simulink model "jielie"  (R2014a)
settings: Solver=ode3  StartTime=0.0  StopTime=200  FixedStep=0.05  RelTol=1e-3
libraries: simulink x8
(part 1 of 3)
settings Model: Creator=Uamoo_15  LastModifiedBy=Administrator
settings DebuggingCC: UnderspecifiedInitializationDetection=Classic  StateNameClashWarn=warning

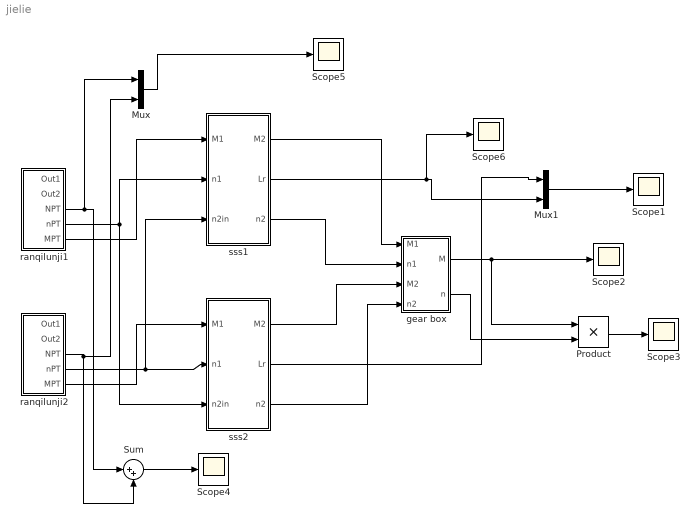
== system jielie ==
  Mux : Mux  Inputs=2
  Mux1 : Mux  Inputs=2
  Product : Product
  Scope{1..6} (6 alike) : Scope
      Scope1 settings: TimeRange=200  YMin=0  YMax=1400  SaveName=ScopeData2
      Scope2 settings: SaveName=ScopeData13
      Scope3 settings: SaveName=ScopeData19
      Scope4 settings: SaveName=ScopeData21
      Scope5 settings: TimeRange=200  YMin=0  YMax=1400  SaveName=ScopeData23
      Scope6 settings: TimeRange=200  YMin=0  YMax=1400  SaveName=ScopeData12
  Sum : Sum  Inputs=|++
  gear box : Subsystem
  ranqilunji1 : Subsystem
  ranqilunji2 : Subsystem
  sss1 : Subsystem
  sss2 : Subsystem
  wires:
  ranqilunji1/4(nPT) -> sss2/3(n2in), sss1/2(n1)
  ranqilunji2/4(nPT) -> sss1/3(n2in), sss2/2(n1)
  ranqilunji1/5(MPT) -> sss1/1(M1)
  ranqilunji2/5(MPT) -> sss2/1(M1)
  sss1/1(M2) -> gear box/1(M1)
  sss2/1(M2) -> gear box/3(M2)
  sss1/3(n2) -> gear box/2(n1)
  sss2/3(n2) -> gear box/4(n2)
  gear box/1(M) -> Product/1, Scope2/1
  gear box/2(n) -> Product/2
  Product/1 -> Scope3/1
  ranqilunji1/3(NPT) -> Mux/1, Sum/1
  ranqilunji2/3(NPT) -> Mux/2, Sum/2
  Sum/1 -> Scope4/1
  Mux/1 -> Scope5/1
  sss1/2(Lr) -> Scope6/1, Mux1/2
  sss2/2(Lr) -> Mux1/1
  Mux1/1 -> Scope1/1

== system jielie/gear box ==
  note: 并车齿轮箱模型
  M1 : Inport
  n1 : Inport  Port=2
  M2 : Inport  Port=3
  n2 : Inport  Port=4
  Add : Sum
  Fcn : Fcn  Expr=1/u
  Gain : Gain  Gain=1/3.5
  Product : Product
  Product1 : Product
  Product2 : Product
  M : Outport
  n : Outport  Port=2
  wires:
  M1/1 -> Product/1
  n1/1 -> Gain/1, Product/2
  Product/1 -> Add/1
  M2/1 -> Product1/1
  n2/1 -> Product1/2
  Product1/1 -> Add/2
  Gain/1 -> n/1, Fcn/1
  Add/1 -> Product2/1
  Fcn/1 -> Product2/2
  Product2/1 -> M/1

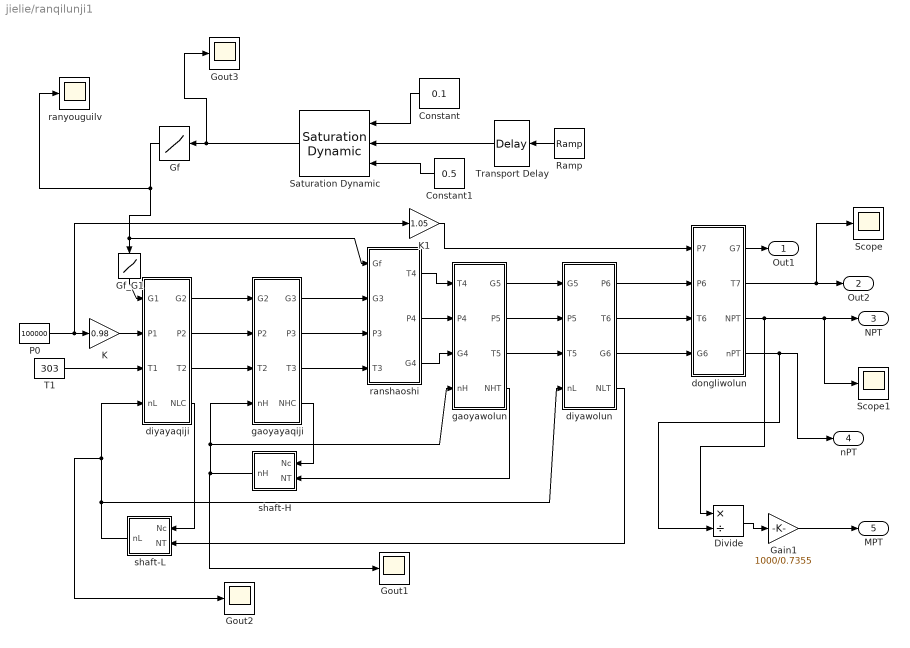
== system jielie/ranqilunji1 ==
  Constant : Constant  Value=0.1
  Constant1 : Constant  Value=0.5
  Divide : Product  Inputs=*/
  Gain1 : Gain  Gain=1000/0.7355
  Gf : Lookup  InputValues=[0,0.03,0.07,0.09,0.11,0.13,0.17,0.2,0.23,0.26,0.28,0.3,0.32,0.34,0.35,0.38,0.4,0.42,0.44,0.47,0.49,0.5,0.52,0.54,0.55,0.59,0.61,0.64,0.66,0.68,0.7,0.72,0.74,0.77,0.81,0.83,0.85,0.88,0.93,0.95,0.97,1]  Table=[0.172,0.236,0.331,0.331,0.366,0.411,0.488,0.536,0.582,0.605,0.644,0.682,0.698,0.728,0.727,0.783,0.783,0.813,0.857,0.886,0.935,0.949,0.95,0.975,0.999,1.022,1.069,1.149,1.153,1.184,1.206,1.233,1.256,1.271,1.325,1.383,1.383,1.439,1.481,1.504,1.52,1.574]
  Gf_G1 : Lookup  InputValues=[0.172,0.236,0.331,0.366,0.411,0.488,0.536,0.582,0.605,0.644,0.682,0.698,0.727,0.728,0.783,0.813,0.857,0.886,0.935,0.949,0.95,0.975,0.999,1.022,1.069,1.149,1.153,1.184,1.206,1.233,1.256,1.271,1.325,1.383,1.439,1.481,1.504,1.52,1.574]  Table="[20.01, 25.93, 38.77,  43.65, 45.94, 51.85, 54.70, 56.85, 59.03, 61.91, 60.44, 61.58, 62.93, 63.04, 65.71,   67.00, 69.52, 70.63, 73.19, 73.46, 73.44, 73.83, 75.62, 76.39, 78.27, 81.17, 81.50, 82.44, 83.44, 84.31, 85.30, 86.17, 87.93, 89.72, 91.51, 93.65, 94.63, 94.92, 97.64]"
  Gout1 : Scope
      settings: TimeRange=10
  Gout2 : Scope
      settings: TimeRange=10  SaveName=ScopeData11
  Gout3 : Scope
      settings: TimeRange=10  SaveName=ScopeData6
  K : Gain  Gain=0.98
  K1 : Gain  Gain=1.05
  P0 : Constant  Value=100000
  Ramp : simulink/Sources/Ramp  slope=1/100  start=0  X0=0.5
  Saturation Dynamic : simulink/Discontinuities/Saturation Dynamic  OutMin=[]  OutMax=[]  OutDataTypeStr=Inherit: Same as second input  OutDataType=fixdt(1, 16)  OutScaling=2^-10  DoSatur=off
  Scope : Scope
      settings: SaveName=ScopeData3
  Scope1 : Scope
      settings: SaveName=ScopeData5
  T1 : Constant  Value=303
  Transport Delay : TransportDelay  DelayTime=40
  diyawolun : Subsystem
  diyayaqiji : Subsystem
  dongliwolun : Subsystem
  gaoyawolun : Subsystem
  gaoyayaqiji : Subsystem
  ranshaoshi : Subsystem
  ranyouguilv : Scope
      settings: TimeRange=10  SaveName=ScopeData8
  shaft-H : Subsystem  mask(rotor module){J=30}
      mask prompts: J "J moment of inertia(Nm)"
      mask help: (pi^2*J*n/900)*(dn/dt)=NT-Nc
  shaft-L : Subsystem  mask(rotor module){J=15}
      mask prompts: J "J moment of inertia(Nm)"
      mask help: (pi^2*J*n/900)*(dn/dt)=NT-Nc
  Out1 : Outport
  Out2 : Outport  Port=2
  NPT : Outport  Port=3
  nPT : Outport  Port=4
  MPT : Outport  Port=5
  wires:
  T1/1 -> diyayaqiji/3(T1)
  K/1 -> diyayaqiji/2(P1)
  diyayaqiji/1(G2) -> gaoyayaqiji/1(G2)
  diyayaqiji/2(P2) -> gaoyayaqiji/2(P2)
  diyayaqiji/3(T2) -> gaoyayaqiji/3(T2)
  gaoyayaqiji/1(G3) -> ranshaoshi/2(G3)
  gaoyayaqiji/2(P3) -> ranshaoshi/3(P3)
  gaoyayaqiji/3(T3) -> ranshaoshi/4(T3)
  gaoyayaqiji/4(NHC) -> shaft-H/1(Nc)
  gaoyawolun/4(NHT) -> shaft-H/2(NT)
  shaft-H/1(nH) -> Gout1/1, gaoyayaqiji/4(nH), gaoyawolun/4(nH)
  diyayaqiji/4(NLC) -> shaft-L/1(Nc)
  diyawolun/4(NLT) -> shaft-L/2(NT)
  Gf_G1/1 -> diyayaqiji/1(G1)
  ranshaoshi/3(G4) -> gaoyawolun/3(G4)
  ranshaoshi/2(P4) -> gaoyawolun/2(P4)
  gaoyawolun/3(T5) -> diyawolun/3(T5)
  gaoyawolun/2(P5) -> diyawolun/2(P5)
  gaoyawolun/1(G5) -> diyawolun/1(G5)
  diyawolun/3(G6) -> dongliwolun/4(G6)
  diyawolun/2(T6) -> dongliwolun/3(T6)
  shaft-L/1(nL) -> diyawolun/4(nL), Gout2/1, diyayaqiji/4(nL)
  diyawolun/1(P6) -> dongliwolun/2(P6)
  P0/1 -> K/1, K1/1
  ranshaoshi/1(T4) -> gaoyawolun/1(T4)
  K1/1 -> dongliwolun/1(P7)
  dongliwolun/1(G7) -> Out1/1
  dongliwolun/2(T7) -> Scope/1, Out2/1
  dongliwolun/3(NPT) -> Divide/1, NPT/1, Scope1/1
  dongliwolun/4(nPT) -> Divide/2, nPT/1
  Constant1/1 -> Saturation Dynamic/3
  Constant/1 -> Saturation Dynamic/1
  Transport Delay/1 -> Saturation Dynamic/2
  Ramp/1 -> Transport Delay/1
  Saturation Dynamic/1 -> Gout3/1, Gf/1
  Gf/1 -> ranyouguilv/1, Gf_G1/1, ranshaoshi/1(Gf)
  Gain1/1 -> MPT/1
  Divide/1 -> Gain1/1

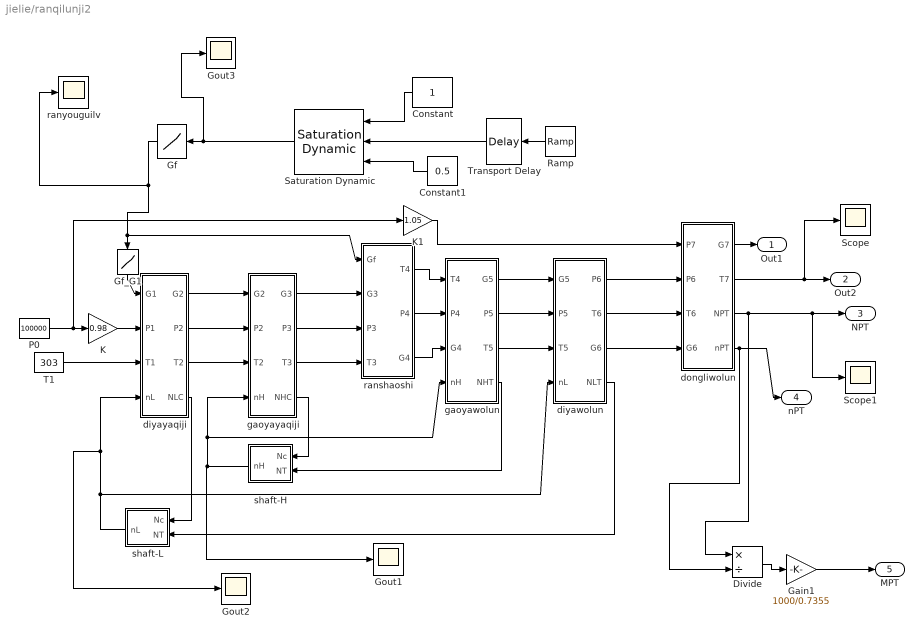
== system jielie/ranqilunji2 ==
  Constant : Constant
  Constant1 : Constant  Value=0.5
  Divide : Product  Inputs=*/
  Gain1 : Gain  Gain=1000/0.7355
  Gf : Lookup  InputValues=[0,0.03,0.07,0.09,0.11,0.13,0.17,0.2,0.23,0.26,0.28,0.3,0.32,0.34,0.35,0.38,0.4,0.42,0.44,0.47,0.49,0.5,0.52,0.54,0.55,0.59,0.61,0.64,0.66,0.68,0.7,0.72,0.74,0.77,0.81,0.83,0.85,0.88,0.93,0.95,0.97,1]  Table=[0.172,0.236,0.331,0.331,0.366,0.411,0.488,0.536,0.582,0.605,0.644,0.682,0.698,0.728,0.727,0.783,0.783,0.813,0.857,0.886,0.935,0.949,0.95,0.975,0.999,1.022,1.069,1.149,1.153,1.184,1.206,1.233,1.256,1.271,1.325,1.383,1.383,1.439,1.481,1.504,1.52,1.574]
  Gf_G1 : Lookup  InputValues=[0.172,0.236,0.331,0.366,0.411,0.488,0.536,0.582,0.605,0.644,0.682,0.698,0.727,0.728,0.783,0.813,0.857,0.886,0.935,0.949,0.95,0.975,0.999,1.022,1.069,1.149,1.153,1.184,1.206,1.233,1.256,1.271,1.325,1.383,1.439,1.481,1.504,1.52,1.574]  Table="[20.01, 25.93, 38.77,  43.65, 45.94, 51.85, 54.70, 56.85, 59.03, 61.91, 60.44, 61.58, 62.93, 63.04, 65.71,   67.00, 69.52, 70.63, 73.19, 73.46, 73.44, 73.83, 75.62, 76.39, 78.27, 81.17, 81.50, 82.44, 83.44, 84.31, 85.30, 86.17, 87.93, 89.72, 91.51, 93.65, 94.63, 94.92, 97.64]"
  Gout1 : Scope
      settings: TimeRange=10
  Gout2 : Scope
      settings: TimeRange=10  SaveName=ScopeData11
  Gout3 : Scope
      settings: TimeRange=10  SaveName=ScopeData6
  K : Gain  Gain=0.98
  K1 : Gain  Gain=1.05
  P0 : Constant  Value=100000
  Ramp : simulink/Sources/Ramp  slope=1/100  start=0  X0=0.5
  Saturation Dynamic : simulink/Discontinuities/Saturation Dynamic  OutMin=[]  OutMax=[]  OutDataTypeStr=Inherit: Same as second input  OutDataType=fixdt(1, 16)  OutScaling=2^-10  DoSatur=off
  Scope : Scope
      settings: SaveName=ScopeData3
  Scope1 : Scope
      settings: SaveName=ScopeData5
  T1 : Constant  Value=303
  Transport Delay : TransportDelay  DelayTime=40
  diyawolun : Subsystem
  diyayaqiji : Subsystem
  dongliwolun : Subsystem
  gaoyawolun : Subsystem
  gaoyayaqiji : Subsystem
  ranshaoshi : Subsystem
  ranyouguilv : Scope
      settings: TimeRange=10  SaveName=ScopeData8
  shaft-H : Subsystem  mask(rotor module){J=30}
      mask prompts: J "J moment of inertia(Nm)"
      mask help: (pi^2*J*n/900)*(dn/dt)=NT-Nc
  shaft-L : Subsystem  mask(rotor module){J=15}
      mask prompts: J "J moment of inertia(Nm)"
      mask help: (pi^2*J*n/900)*(dn/dt)=NT-Nc
  Out1 : Outport
  Out2 : Outport  Port=2
  NPT : Outport  Port=3
  nPT : Outport  Port=4
  MPT : Outport  Port=5
  wires:
  T1/1 -> diyayaqiji/3(T1)
  K/1 -> diyayaqiji/2(P1)
  diyayaqiji/1(G2) -> gaoyayaqiji/1(G2)
  diyayaqiji/2(P2) -> gaoyayaqiji/2(P2)
  diyayaqiji/3(T2) -> gaoyayaqiji/3(T2)
  gaoyayaqiji/1(G3) -> ranshaoshi/2(G3)
  gaoyayaqiji/2(P3) -> ranshaoshi/3(P3)
  gaoyayaqiji/3(T3) -> ranshaoshi/4(T3)
  gaoyayaqiji/4(NHC) -> shaft-H/1(Nc)
  gaoyawolun/4(NHT) -> shaft-H/2(NT)
  shaft-H/1(nH) -> Gout1/1, gaoyayaqiji/4(nH), gaoyawolun/4(nH)
  diyayaqiji/4(NLC) -> shaft-L/1(Nc)
  diyawolun/4(NLT) -> shaft-L/2(NT)
  Gf_G1/1 -> diyayaqiji/1(G1)
  ranshaoshi/3(G4) -> gaoyawolun/3(G4)
  ranshaoshi/2(P4) -> gaoyawolun/2(P4)
  gaoyawolun/3(T5) -> diyawolun/3(T5)
  gaoyawolun/2(P5) -> diyawolun/2(P5)
  gaoyawolun/1(G5) -> diyawolun/1(G5)
  diyawolun/3(G6) -> dongliwolun/4(G6)
  diyawolun/2(T6) -> dongliwolun/3(T6)
  shaft-L/1(nL) -> diyawolun/4(nL), Gout2/1, diyayaqiji/4(nL)
  diyawolun/1(P6) -> dongliwolun/2(P6)
  P0/1 -> K/1, K1/1
  ranshaoshi/1(T4) -> gaoyawolun/1(T4)
  K1/1 -> dongliwolun/1(P7)
  dongliwolun/1(G7) -> Out1/1
  dongliwolun/2(T7) -> Scope/1, Out2/1
  dongliwolun/3(NPT) -> Divide/1, NPT/1, Scope1/1
  dongliwolun/4(nPT) -> Divide/2, nPT/1
  Constant1/1 -> Saturation Dynamic/3
  Constant/1 -> Saturation Dynamic/1
  Transport Delay/1 -> Saturation Dynamic/2
  Ramp/1 -> Transport Delay/1
  Saturation Dynamic/1 -> Gout3/1, Gf/1
  Gf/1 -> ranyouguilv/1, Gf_G1/1, ranshaoshi/1(Gf)
  Gain1/1 -> MPT/1
  Divide/1 -> Gain1/1

== system jielie/sss1 ==
  note: sss离合器模块
  M1 : Inport
  n1 : Inport  Port=2
  n2in : Inport  Port=3
  Add : Sum  Inputs=+-
  Clock : Clock
  Constant : Constant  Value=15
  Fcn : Fcn  Expr=u*pi/30
  Subsystem : Subsystem
  Subsystem1 : Subsystem
  Subsystem2 : Subsystem
  Subsystem3 : Subsystem
  Switch : Switch
  Switch1 : Switch  Threshold=40
  M2 : Outport
  Lr : Outport  Port=2
  n2 : Outport  Port=3
  wires:
  Fcn/1 -> Add/2
  Switch/1 -> n2/1
  M1/1 -> Subsystem3/1(M1)
  Subsystem/1(J1) -> Subsystem3/3(J1)
  Subsystem/2(Jz) -> Subsystem1/2(Jz)
  Subsystem3/1(Mfzf) -> Subsystem1/1(Mfzf)
  Subsystem3/3(C1) -> Subsystem1/3(C1)
  Subsystem1/1(Mr) -> Subsystem2/1(Mr)
  Subsystem1/3(C2) -> Subsystem2/3(C2)
  Subsystem1/2(Lr) -> Switch1/1, Switch/2
  Subsystem3/2(wf) -> Add/1
  Subsystem/3(J2) -> Subsystem2/2(J2)
  Subsystem2/1(M2) -> M2/1
  Subsystem/4(f) -> Subsystem1/4(f)
  n2in/1 -> Subsystem2/4(n2in)
  Add/1 -> Subsystem1/5(Wz)
  Subsystem2/2(n2) -> Fcn/1, Switch/3
  n1/1 -> Subsystem3/2(n1), Switch/1
  Constant/1 -> Switch1/3
  Switch1/1 -> Lr/1
  Clock/1 -> Switch1/2

== system jielie/sss2 ==
  note: sss离合器模块
  M1 : Inport
  n1 : Inport  Port=2
  n2in : Inport  Port=3
  Add : Sum  Inputs=+-
  Clock : Clock
  Constant : Constant  Value=15
  Fcn : Fcn  Expr=u*pi/30
  Subsystem : Subsystem
  Subsystem1 : Subsystem
  Subsystem2 : Subsystem
  Subsystem3 : Subsystem
  Switch : Switch
  Switch1 : Switch  Threshold=40
  M2 : Outport
  Lr : Outport  Port=2
  n2 : Outport  Port=3
  wires:
  Fcn/1 -> Add/2
  Switch/1 -> n2/1
  M1/1 -> Subsystem3/1(M1)
  Subsystem/1(J1) -> Subsystem3/3(J1)
  Subsystem/2(Jz) -> Subsystem1/2(Jz)
  Subsystem3/1(Mfzf) -> Subsystem1/1(Mfzf)
  Subsystem3/3(C1) -> Subsystem1/3(C1)
  Subsystem1/1(Mr) -> Subsystem2/1(Mr)
  Subsystem1/3(C2) -> Subsystem2/3(C2)
  Subsystem3/2(wf) -> Add/1
  Subsystem/3(J2) -> Subsystem2/2(J2)
  Subsystem2/1(M2) -> M2/1
  Subsystem/4(f) -> Subsystem1/4(f)
  n2in/1 -> Subsystem2/4(n2in)
  Add/1 -> Subsystem1/5(Wz)
  Subsystem2/2(n2) -> Fcn/1, Switch/3
  n1/1 -> Subsystem3/2(n1), Switch/1
  Subsystem1/2(Lr) -> Switch1/1, Switch/2
  Clock/1 -> Switch1/2
  Constant/1 -> Switch1/3
  Switch1/1 -> Lr/1

== system jielie/ranqilunji1/diyawolun ==
  G5 : Inport
  P5 : Inport  Port=2
  T5 : Inport  Port=3
  nL : Inport  Port=4
  Divide : Product  Inputs=*/
  Scope1 : Scope
      settings: TimeRange=100  YMin=5000  YMax=25000  SaveName=ScopeData28
  Scope2 : Scope
      settings: TimeRange=100  YMin=5000  YMax=25000  SaveName=ScopeData4
  Scope3 : Scope
      settings: TimeRange=100  YMin=5000  YMax=25000  SaveName=ScopeData20
  n1-p6 : Lookup  InputValues=[2849,4651,4850,5410,5586,5742,6024,6092,6102,6211,6385,6425,6435,6609,6698,6732,7015,7080,7185]  Table=[113000,150000,157000,180000,190000,201000,221000,229000,229500,242000,267000,272000,277000,306000,321000,322000,354000,360000,371000]
  n2-etaH : Lookup  InputValues=[4300 5000 5500 6000 6500 7000 7500 8000 9000 9500]  Table=[0.82 0.83 0.835 0.84 0.85 0.86 0.875 0.87 0.865 0.86]
  turbine_TN : Subsystem  mask(Turbine_Tout Nout module){}
  P6 : Outport
  T6 : Outport  Port=2
  G6 : Outport  Port=3
  NLT : Outport  Port=4
  wires:
  n2-etaH/1 -> turbine_TN/2(eta)
  P5/1 -> Divide/1
  nL/1 -> n2-etaH/1, n1-p6/1
  turbine_TN/1(Tout) -> T6/1, Scope2/1
  T5/1 -> turbine_TN/3(Tin)
  turbine_TN/2(Nout) -> NLT/1
  G5/1 -> turbine_TN/4(Gin), G6/1
  n1-p6/1 -> Divide/2, P6/1, Scope1/1
  Divide/1 -> turbine_TN/1(Pi), Scope3/1

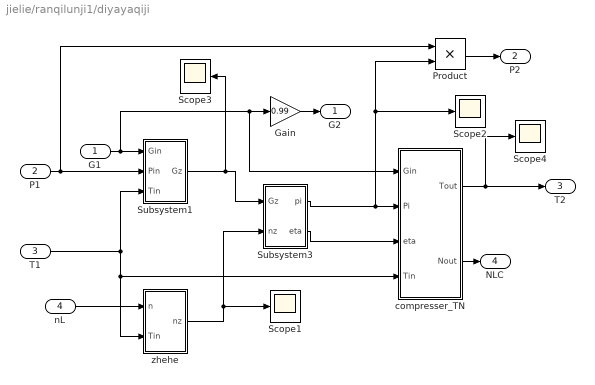
== system jielie/ranqilunji1/diyayaqiji ==
  G1 : Inport
  P1 : Inport  Port=2
  T1 : Inport  Port=3
  nL : Inport  Port=4
  Gain : Gain  Gain=0.99
  Product : Product  RndMeth=Zero
  Scope{1..4} (4 alike) : Scope
      Scope1 settings: YMin=2829.54  YMax=3127.38  SaveName=ScopeData14
      Scope2 settings: YMin=2829.54  YMax=3127.38  SaveName=ScopeData9
      Scope3 settings: YMin=2829.54  YMax=3127.38  SaveName=ScopeData30
      Scope4 settings: TimeRange=80  YMin=5000  YMax=30000  SaveName=ScopeData32
  Subsystem1 : Subsystem
  Subsystem3 : Subsystem
  compresser_TN : Subsystem  mask(Compressor_Tout Nout module){}
  zhehe : Subsystem
  G2 : Outport
  P2 : Outport  Port=2
  T2 : Outport  Port=3
  NLC : Outport  Port=4
  wires:
  Subsystem3/1(pi) -> compresser_TN/2(Pi), Product/2, Scope2/1
  Subsystem3/2(eta) -> compresser_TN/3(eta)
  T1/1 -> zhehe/2(Tin), compresser_TN/4(Tin), Subsystem1/3(Tin)
  Gain/1 -> G2/1
  compresser_TN/1(Tout) -> T2/1, Scope4/1
  compresser_TN/2(Nout) -> NLC/1
  Subsystem1/1(Gz) -> Scope3/1, Subsystem3/1(Gz)
  G1/1 -> Subsystem1/1(Gin), Gain/1, compresser_TN/1(Gin)
  P1/1 -> Subsystem1/2(Pin), Product/1
  Product/1 -> P2/1
  nL/1 -> zhehe/1(n)
  zhehe/1(nz) -> Scope1/1, Subsystem3/2(nz)

== system jielie/ranqilunji1/dongliwolun ==
  P7 : Inport
  P6 : Inport  Port=2
  T6 : Inport  Port=3
  G6 : Inport  Port=4
  Divide : Product  Inputs=*/
  Pi-eta1 : Lookup  InputValues=[1,1.11 1.41 1.51 1.81 2.0 2.21 2.41 2.61 2.81]  Table=[0.825,0.83 0.85 0.86 0.88 0.90 0.905 0.91 0.905 0.9]
  Pi-eta2 : Lookup  InputValues=[307,625,1634,2141,2611,3121,4030,4941,5687,6256,6755,7309,7716,8175,8374,9153,9719,10196,10702,11284,11832,12033,12512,13051,13298,14334,14778,15580,16003,16531,16669,17381,17948,18600,19648,20212,20613,21462,22525,23139,23520,24372]  Table=[878,1243,1778,1749,1547,1574,1765,1930,2049,2045,2069,2150,2158,2185,2214,2272,2274,2209,2231,2240,2252,2500,2569,2649,2574,2650,2617,2639,2697,2653,2702,2785,2901,2979,3042,2919,2951,3108,3089,3056,3065,3142]
  Scope6 : Scope
      settings: YMin=2829.54  YMax=3127.38  SaveName=ScopeData22
  turbine_TN : Subsystem  mask(Turbine_Tout Nout module){}
  G7 : Outport
  T7 : Outport  Port=2
  NPT : Outport  Port=3
  nPT : Outport  Port=4
  wires:
  turbine_TN/1(Tout) -> T7/1
  turbine_TN/2(Nout) -> NPT/1, Pi-eta2/1
  G6/1 -> turbine_TN/3(Gin), G7/1
  Divide/1 -> Scope6/1, turbine_TN/1(Pi), Pi-eta1/1
  T6/1 -> turbine_TN/4(Tin)
  Pi-eta1/1 -> turbine_TN/2(eta)
  P6/1 -> Divide/1
  P7/1 -> Divide/2
  Pi-eta2/1 -> nPT/1

== system jielie/ranqilunji1/gaoyawolun ==
  T4 : Inport
  P4 : Inport  Port=2
  G4 : Inport  Port=3
  nH : Inport  Port=4
  Divide : Product  Inputs=*/
  Scope3 : Scope
      settings: TimeRange=100  YMin=5000  YMax=25000  SaveName=ScopeData34
  n2-etaH : Lookup  InputValues=[6000 6300 6500 6800 7000 7150 7300 7500 7800]  Table=[0.81 0.83 0.85 0.87 0.88 0.87 0.86 0.855 0.85]
  n2-p5 : Lookup  InputValues=[5832,7212,7282,7644,7752,7853,8033,8092 8211 8392 8430 8452 8670 8767 8960 8999 9073]  Table=[154000,269000,296000,361000,391000,419000,476000,494000 534000 596000 609000 616000 684000 719000 806000 814000 831000]
  pi : Scope
      settings: TimeRange=100  YMin=2829.54  YMax=3127.38  SaveName=ScopeData17
  pi1 : Scope
      settings: TimeRange=100  YMin=2829.54  YMax=3127.38  SaveName=ScopeData7
  pi2 : Scope
      settings: TimeRange=100  YMin=2829.54  YMax=3127.38  SaveName=ScopeData35
  turbine_TN : Subsystem  mask(Turbine_Tout Nout module){}
  G5 : Outport
  P5 : Outport  Port=2
  T5 : Outport  Port=3
  NHT : Outport  Port=4
  wires:
  n2-etaH/1 -> turbine_TN/2(eta)
  P4/1 -> Divide/1
  nH/1 -> pi2/1, n2-etaH/1, n2-p5/1
  turbine_TN/1(Tout) -> T5/1, pi1/1
  T4/1 -> turbine_TN/3(Tin)
  turbine_TN/2(Nout) -> NHT/1
  G4/1 -> turbine_TN/4(Gin), G5/1
  Divide/1 -> turbine_TN/1(Pi), pi/1
  n2-p5/1 -> Divide/2, P5/1, Scope3/1

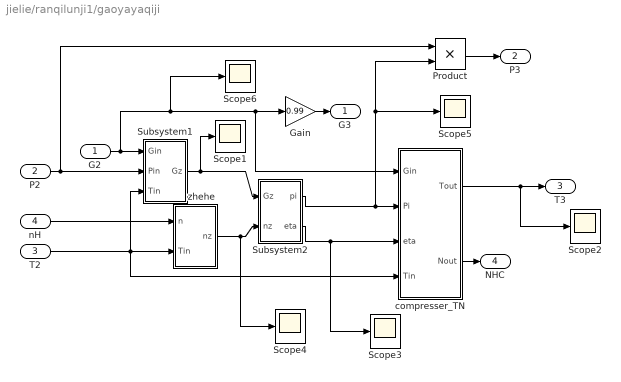
== system jielie/ranqilunji1/gaoyayaqiji ==
  G2 : Inport
  P2 : Inport  Port=2
  T2 : Inport  Port=3
  nH : Inport  Port=4
  Gain : Gain  Gain=0.99
  Product : Product  RndMeth=Zero
  Scope{1..6} (6 alike) : Scope
      Scope1 settings: YMin=2829.54  YMax=3127.38  SaveName=ScopeData16
      Scope2 settings: YMin=2829.54  YMax=3127.38  SaveName=ScopeData29
      Scope3 settings: YMin=2829.54  YMax=3127.38  SaveName=ScopeData24
      Scope4 settings: YMin=2829.54  YMax=3127.38  SaveName=ScopeData31
      Scope5 settings: YMin=2829.54  YMax=3127.38  SaveName=ScopeData10
      Scope6 settings: YMin=2829.54  YMax=3127.38  SaveName=ScopeData15
  Subsystem1 : Subsystem
  Subsystem2 : Subsystem
  compresser_TN : Subsystem  mask(Compressor_Tout Nout module){}
  zhehe : Subsystem
  G3 : Outport
  P3 : Outport  Port=2
  T3 : Outport  Port=3
  NHC : Outport  Port=4
  wires:
  zhehe/1(nz) -> Scope4/1, Subsystem2/2(nz)
  Subsystem2/1(pi) -> compresser_TN/2(Pi), Product/2, Scope5/1
  Subsystem2/2(eta) -> compresser_TN/3(eta), Scope3/1
  T2/1 -> zhehe/2(Tin), compresser_TN/4(Tin), Subsystem1/3(Tin)
  nH/1 -> zhehe/1(n)
  Gain/1 -> G3/1
  compresser_TN/1(Tout) -> T3/1, Scope2/1
  compresser_TN/2(Nout) -> NHC/1
  Subsystem1/1(Gz) -> Scope1/1, Subsystem2/1(Gz)
  G2/1 -> Subsystem1/1(Gin), Gain/1, compresser_TN/1(Gin), Scope6/1
  P2/1 -> Subsystem1/2(Pin), Product/1
  Product/1 -> P3/1

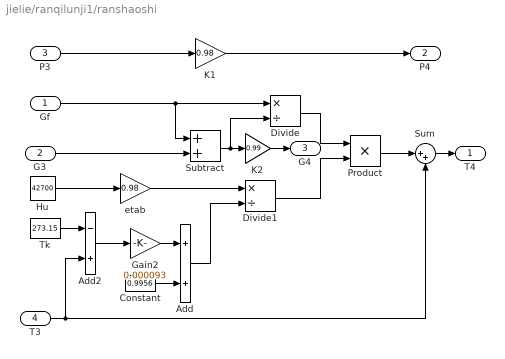
== system jielie/ranqilunji1/ranshaoshi ==
  Gf : Inport
  G3 : Inport  Port=2
  P3 : Inport  Port=3
  T3 : Inport  Port=4
  Add : Sum
  Add2 : Sum  Inputs=-+
  Constant : Constant  Value=0.9956
  Divide : Product  Inputs=*/
  Divide1 : Product  Inputs=*/
  Gain2 : Gain  Gain=0.000093
  Hu : Constant  Value=42700
  K1 : Gain  Gain=0.98
  K2 : Gain  Gain=0.99
  Product : Product  RndMeth=Zero
  Subtract : Sum
  Sum : Sum  Inputs=|++
  Tk : Constant  Value=273.15
  etab : Gain  Gain=0.98
  T4 : Outport
  P4 : Outport  Port=2
  G4 : Outport  Port=3
  wires:
  Gf/1 -> Divide/1, Subtract/1
  Divide/1 -> Product/1
  G3/1 -> Subtract/2
  Subtract/1 -> Divide/2, K2/1
  Hu/1 -> etab/1
  etab/1 -> Divide1/1
  Divide1/1 -> Product/2
  Product/1 -> Sum/1
  Sum/1 -> T4/1
  T3/1 -> Add2/2, Sum/2
  P3/1 -> K1/1
  K1/1 -> P4/1
  Constant/1 -> Add/2
  Gain2/1 -> Add/1
  Tk/1 -> Add2/1
  Add2/1 -> Gain2/1
  Add/1 -> Divide1/2
  K2/1 -> G4/1

== system jielie/ranqilunji1/shaft-H ==
  Nc : Inport
  NT : Inport  Port=2
  Add : Sum  Inputs=-+
  Divide : Product  Inputs=3
  Fcn : Fcn  Expr=1/u
  Fcn1 : Fcn  Expr=1/u
  Gain : Gain  Gain=15/(pi*pi)
  Gain3 : Gain  Gain=60
  Integrator : Integrator  InitialCondition=143.58
  J : Constant  Value=J
  nH : Outport
  wires:
  Nc/1 -> Add/1
  NT/1 -> Add/2
  Divide/1 -> Integrator/1
  Integrator/1 -> Fcn1/1, Gain3/1
  Add/1 -> Divide/1
  J/1 -> Fcn/1
  Gain/1 -> Divide/2
  Fcn/1 -> Gain/1
  Fcn1/1 -> Divide/3
  Gain3/1 -> nH/1

== system jielie/ranqilunji1/shaft-L ==
  Nc : Inport
  NT : Inport  Port=2
  Add : Sum  Inputs=-+
  Constant : Constant  Value=0.93
  Constant1 : Constant  Value=0.3
  Divide : Product  Inputs=3
  Fcn : Fcn  Expr=1/u
  Fcn1 : Fcn  Expr=1/u
  Gain : Gain  Gain=15/(pi*pi)
  Gain2 : Gain  Gain=60
  Integrator : Integrator  InitialCondition=105.9
  J : Constant  Value=J
  Ramp : simulink/Sources/Ramp  slope=1/100  start=0  X0=0.3
  Saturation Dynamic : simulink/Discontinuities/Saturation Dynamic  OutMin=[]  OutMax=[]  OutDataTypeStr=Inherit: Same as second input  OutDataType=fixdt(1, 16)  OutScaling=2^-10  DoSatur=off
  Scope : Scope
  Transport Delay : TransportDelay  DelayTime=20
  nL : Outport
  wires:
  Nc/1 -> Add/1
  NT/1 -> Add/2
  Divide/1 -> Integrator/1
  Integrator/1 -> Fcn1/1, Gain2/1
  Add/1 -> Divide/1
  J/1 -> Fcn/1
  Gain/1 -> Divide/2
  Fcn/1 -> Gain/1
  Fcn1/1 -> Divide/3
  Gain2/1 -> nL/1, Scope/1
  Constant1/1 -> Saturation Dynamic/3
  Constant/1 -> Saturation Dynamic/1
  Transport Delay/1 -> Saturation Dynamic/2
  Ramp/1 -> Transport Delay/1

== system jielie/ranqilunji2/diyawolun ==
  G5 : Inport
  P5 : Inport  Port=2
  T5 : Inport  Port=3
  nL : Inport  Port=4
  Divide : Product  Inputs=*/
  Scope1 : Scope
      settings: TimeRange=100  YMin=5000  YMax=25000  SaveName=ScopeData28
  Scope2 : Scope
      settings: TimeRange=100  YMin=5000  YMax=25000  SaveName=ScopeData4
  Scope3 : Scope
      settings: TimeRange=100  YMin=5000  YMax=25000  SaveName=ScopeData20
  n1-p6 : Lookup  InputValues=[2849,4651,4850,5410,5586,5742,6024,6092,6102,6211,6385,6425,6435,6609,6698,6732,7015,7080,7185]  Table=[113000,150000,157000,180000,190000,201000,221000,229000,229500,242000,267000,272000,277000,306000,321000,322000,354000,360000,371000]
  n2-etaH : Lookup  InputValues=[4300 5000 5500 6000 6500 7000 7500 8000 9000 9500]  Table=[0.82 0.83 0.835 0.84 0.85 0.86 0.875 0.87 0.865 0.86]
  turbine_TN : Subsystem  mask(Turbine_Tout Nout module){}
  P6 : Outport
  T6 : Outport  Port=2
  G6 : Outport  Port=3
  NLT : Outport  Port=4
  wires:
  n2-etaH/1 -> turbine_TN/2(eta)
  P5/1 -> Divide/1
  nL/1 -> n2-etaH/1, n1-p6/1
  turbine_TN/1(Tout) -> T6/1, Scope2/1
  T5/1 -> turbine_TN/3(Tin)
  turbine_TN/2(Nout) -> NLT/1
  G5/1 -> turbine_TN/4(Gin), G6/1
  n1-p6/1 -> Divide/2, P6/1, Scope1/1
  Divide/1 -> turbine_TN/1(Pi), Scope3/1

== system jielie/ranqilunji2/diyayaqiji ==
  G1 : Inport
  P1 : Inport  Port=2
  T1 : Inport  Port=3
  nL : Inport  Port=4
  Gain : Gain  Gain=0.99
  Product : Product  RndMeth=Zero
  Scope{1..4} (4 alike) : Scope
      Scope1 settings: YMin=2829.54  YMax=3127.38  SaveName=ScopeData14
      Scope2 settings: YMin=2829.54  YMax=3127.38  SaveName=ScopeData9
      Scope3 settings: YMin=2829.54  YMax=3127.38  SaveName=ScopeData30
      Scope4 settings: TimeRange=80  YMin=5000  YMax=30000  SaveName=ScopeData32
  Subsystem1 : Subsystem
  Subsystem3 : Subsystem
  compresser_TN : Subsystem  mask(Compressor_Tout Nout module){}
  zhehe : Subsystem
  G2 : Outport
  P2 : Outport  Port=2
  T2 : Outport  Port=3
  NLC : Outport  Port=4
  wires:
  Subsystem3/1(pi) -> compresser_TN/2(Pi), Product/2, Scope2/1
  Subsystem3/2(eta) -> compresser_TN/3(eta)
  T1/1 -> zhehe/2(Tin), compresser_TN/4(Tin), Subsystem1/3(Tin)
  Gain/1 -> G2/1
  compresser_TN/1(Tout) -> T2/1, Scope4/1
  compresser_TN/2(Nout) -> NLC/1
  Subsystem1/1(Gz) -> Scope3/1, Subsystem3/1(Gz)
  G1/1 -> Subsystem1/1(Gin), Gain/1, compresser_TN/1(Gin)
  P1/1 -> Subsystem1/2(Pin), Product/1
  Product/1 -> P2/1
  nL/1 -> zhehe/1(n)
  zhehe/1(nz) -> Scope1/1, Subsystem3/2(nz)

== system jielie/ranqilunji2/dongliwolun ==
  P7 : Inport
  P6 : Inport  Port=2
  T6 : Inport  Port=3
  G6 : Inport  Port=4
  Divide : Product  Inputs=*/
  Pi-eta1 : Lookup  InputValues=[1,1.11 1.41 1.51 1.81 2.0 2.21 2.41 2.61 2.81]  Table=[0.825,0.83 0.85 0.86 0.88 0.90 0.905 0.91 0.905 0.9]
  Pi-eta2 : Lookup  InputValues=[307,625,1634,2141,2611,3121,4030,4941,5687,6256,6755,7309,7716,8175,8374,9153,9719,10196,10702,11284,11832,12033,12512,13051,13298,14334,14778,15580,16003,16531,16669,17381,17948,18600,19648,20212,20613,21462,22525,23139,23520,24372]  Table=[878,1243,1778,1749,1547,1574,1765,1930,2049,2045,2069,2150,2158,2185,2214,2272,2274,2209,2231,2240,2252,2500,2569,2649,2574,2650,2617,2639,2697,2653,2702,2785,2901,2979,3042,2919,2951,3108,3089,3056,3065,3142]
  Scope6 : Scope
      settings: YMin=2829.54  YMax=3127.38  SaveName=ScopeData22
  turbine_TN : Subsystem  mask(Turbine_Tout Nout module){}
  G7 : Outport
  T7 : Outport  Port=2
  NPT : Outport  Port=3
  nPT : Outport  Port=4
  wires:
  turbine_TN/1(Tout) -> T7/1
  turbine_TN/2(Nout) -> NPT/1, Pi-eta2/1
  G6/1 -> turbine_TN/3(Gin), G7/1
  Divide/1 -> Scope6/1, turbine_TN/1(Pi), Pi-eta1/1
  T6/1 -> turbine_TN/4(Tin)
  Pi-eta1/1 -> turbine_TN/2(eta)
  P6/1 -> Divide/1
  P7/1 -> Divide/2
  Pi-eta2/1 -> nPT/1

== system jielie/ranqilunji2/gaoyawolun ==
  T4 : Inport
  P4 : Inport  Port=2
  G4 : Inport  Port=3
  nH : Inport  Port=4
  Divide : Product  Inputs=*/
  Scope3 : Scope
      settings: TimeRange=100  YMin=5000  YMax=25000  SaveName=ScopeData34
  n2-etaH : Lookup  InputValues=[6000 6300 6500 6800 7000 7150 7300 7500 7800]  Table=[0.81 0.83 0.85 0.87 0.88 0.87 0.86 0.855 0.85]
  n2-p5 : Lookup  InputValues=[5832,7212,7282,7644,7752,7853,8033,8092 8211 8392 8430 8452 8670 8767 8960 8999 9073]  Table=[154000,269000,296000,361000,391000,419000,476000,494000 534000 596000 609000 616000 684000 719000 806000 814000 831000]
  pi : Scope
      settings: TimeRange=100  YMin=2829.54  YMax=3127.38  SaveName=ScopeData17
  pi1 : Scope
      settings: TimeRange=100  YMin=2829.54  YMax=3127.38  SaveName=ScopeData7
  pi2 : Scope
      settings: TimeRange=100  YMin=2829.54  YMax=3127.38  SaveName=ScopeData35
  turbine_TN : Subsystem  mask(Turbine_Tout Nout module){}
  G5 : Outport
  P5 : Outport  Port=2
  T5 : Outport  Port=3
  NHT : Outport  Port=4
  wires:
  n2-etaH/1 -> turbine_TN/2(eta)
  P4/1 -> Divide/1
  nH/1 -> pi2/1, n2-etaH/1, n2-p5/1
  turbine_TN/1(Tout) -> T5/1, pi1/1
  T4/1 -> turbine_TN/3(Tin)
  turbine_TN/2(Nout) -> NHT/1
  G4/1 -> turbine_TN/4(Gin), G5/1
  Divide/1 -> turbine_TN/1(Pi), pi/1
  n2-p5/1 -> Divide/2, P5/1, Scope3/1

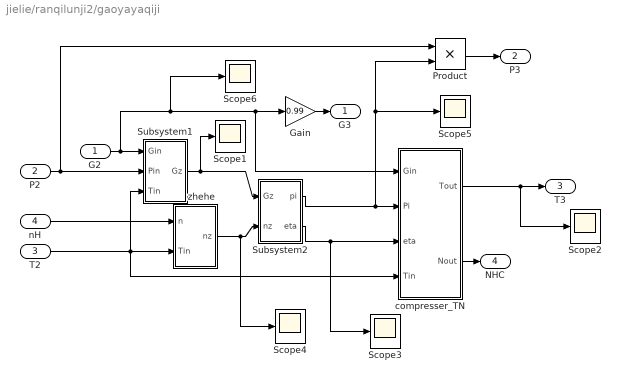
== system jielie/ranqilunji2/gaoyayaqiji ==
  G2 : Inport
  P2 : Inport  Port=2
  T2 : Inport  Port=3
  nH : Inport  Port=4
  Gain : Gain  Gain=0.99
  Product : Product  RndMeth=Zero
  Scope{1..6} (6 alike) : Scope
      Scope1 settings: YMin=2829.54  YMax=3127.38  SaveName=ScopeData16
      Scope2 settings: YMin=2829.54  YMax=3127.38  SaveName=ScopeData29
      Scope3 settings: YMin=2829.54  YMax=3127.38  SaveName=ScopeData24
      Scope4 settings: YMin=2829.54  YMax=3127.38  SaveName=ScopeData31
      Scope5 settings: YMin=2829.54  YMax=3127.38  SaveName=ScopeData10
      Scope6 settings: YMin=2829.54  YMax=3127.38  SaveName=ScopeData15
  Subsystem1 : Subsystem
  Subsystem2 : Subsystem
  compresser_TN : Subsystem  mask(Compressor_Tout Nout module){}
  zhehe : Subsystem
  G3 : Outport
  P3 : Outport  Port=2
  T3 : Outport  Port=3
  NHC : Outport  Port=4
  wires:
  zhehe/1(nz) -> Scope4/1, Subsystem2/2(nz)
  Subsystem2/1(pi) -> compresser_TN/2(Pi), Product/2, Scope5/1
  Subsystem2/2(eta) -> compresser_TN/3(eta), Scope3/1
  T2/1 -> zhehe/2(Tin), compresser_TN/4(Tin), Subsystem1/3(Tin)
  nH/1 -> zhehe/1(n)
  Gain/1 -> G3/1
  compresser_TN/1(Tout) -> T3/1, Scope2/1
  compresser_TN/2(Nout) -> NHC/1
  Subsystem1/1(Gz) -> Scope1/1, Subsystem2/1(Gz)
  G2/1 -> Subsystem1/1(Gin), Gain/1, compresser_TN/1(Gin), Scope6/1
  P2/1 -> Subsystem1/2(Pin), Product/1
  Product/1 -> P3/1

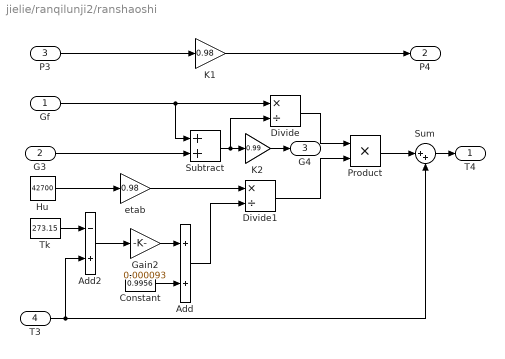
== system jielie/ranqilunji2/ranshaoshi ==
  Gf : Inport
  G3 : Inport  Port=2
  P3 : Inport  Port=3
  T3 : Inport  Port=4
  Add : Sum
  Add2 : Sum  Inputs=-+
  Constant : Constant  Value=0.9956
  Divide : Product  Inputs=*/
  Divide1 : Product  Inputs=*/
  Gain2 : Gain  Gain=0.000093
  Hu : Constant  Value=42700
  K1 : Gain  Gain=0.98
  K2 : Gain  Gain=0.99
  Product : Product  RndMeth=Zero
  Subtract : Sum
  Sum : Sum  Inputs=|++
  Tk : Constant  Value=273.15
  etab : Gain  Gain=0.98
  T4 : Outport
  P4 : Outport  Port=2
  G4 : Outport  Port=3
  wires:
  Gf/1 -> Divide/1, Subtract/1
  Divide/1 -> Product/1
  G3/1 -> Subtract/2
  Subtract/1 -> Divide/2, K2/1
  Hu/1 -> etab/1
  etab/1 -> Divide1/1
  Divide1/1 -> Product/2
  Product/1 -> Sum/1
  Sum/1 -> T4/1
  T3/1 -> Add2/2, Sum/2
  P3/1 -> K1/1
  K1/1 -> P4/1
  Constant/1 -> Add/2
  Gain2/1 -> Add/1
  Tk/1 -> Add2/1
  Add2/1 -> Gain2/1
  Add/1 -> Divide1/2
  K2/1 -> G4/1

== system jielie/ranqilunji2/shaft-H ==
  Nc : Inport
  NT : Inport  Port=2
  Add : Sum  Inputs=-+
  Divide : Product  Inputs=3
  Fcn : Fcn  Expr=1/u
  Fcn1 : Fcn  Expr=1/u
  Gain : Gain  Gain=15/(pi*pi)
  Gain3 : Gain  Gain=60
  Integrator : Integrator  InitialCondition=143.58
  J : Constant  Value=J
  nH : Outport
  wires:
  Nc/1 -> Add/1
  NT/1 -> Add/2
  Divide/1 -> Integrator/1
  Integrator/1 -> Fcn1/1, Gain3/1
  Add/1 -> Divide/1
  J/1 -> Fcn/1
  Gain/1 -> Divide/2
  Fcn/1 -> Gain/1
  Fcn1/1 -> Divide/3
  Gain3/1 -> nH/1

== system jielie/ranqilunji2/shaft-L ==
  Nc : Inport
  NT : Inport  Port=2
  Add : Sum  Inputs=-+
  Constant : Constant  Value=0.93
  Constant1 : Constant  Value=0.3
  Divide : Product  Inputs=3
  Fcn : Fcn  Expr=1/u
  Fcn1 : Fcn  Expr=1/u
  Gain : Gain  Gain=15/(pi*pi)
  Gain2 : Gain  Gain=60
  Integrator : Integrator  InitialCondition=105.9
  J : Constant  Value=J
  Ramp : simulink/Sources/Ramp  slope=1/100  start=0  X0=0.3
  Saturation Dynamic : simulink/Discontinuities/Saturation Dynamic  OutMin=[]  OutMax=[]  OutDataTypeStr=Inherit: Same as second input  OutDataType=fixdt(1, 16)  OutScaling=2^-10  DoSatur=off
  Scope : Scope
  Transport Delay : TransportDelay  DelayTime=20
  nL : Outport
  wires:
  Nc/1 -> Add/1
  NT/1 -> Add/2
  Divide/1 -> Integrator/1
  Integrator/1 -> Fcn1/1, Gain2/1
  Add/1 -> Divide/1
  J/1 -> Fcn/1
  Gain/1 -> Divide/2
  Fcn/1 -> Gain/1
  Fcn1/1 -> Divide/3
  Gain2/1 -> nL/1, Scope/1
  Constant1/1 -> Saturation Dynamic/3
  Constant/1 -> Saturation Dynamic/1
  Transport Delay/1 -> Saturation Dynamic/2
  Ramp/1 -> Transport Delay/1

== system jielie/sss1/Subsystem ==
  note: 阻尼系数模块
  J : Constant  Value=0.119507
  J2l : Constant  Value=0.092495
  Jk : Constant  Value=0.0694875
  f1 : Constant  Value=0.6
  J1 : Outport
  Jz : Outport  Port=2
  J2 : Outport  Port=3
  f : Outport  Port=4
  wires:
  J/1 -> J1/1
  Jk/1 -> Jz/1
  J2l/1 -> J2/1
  f1/1 -> f/1

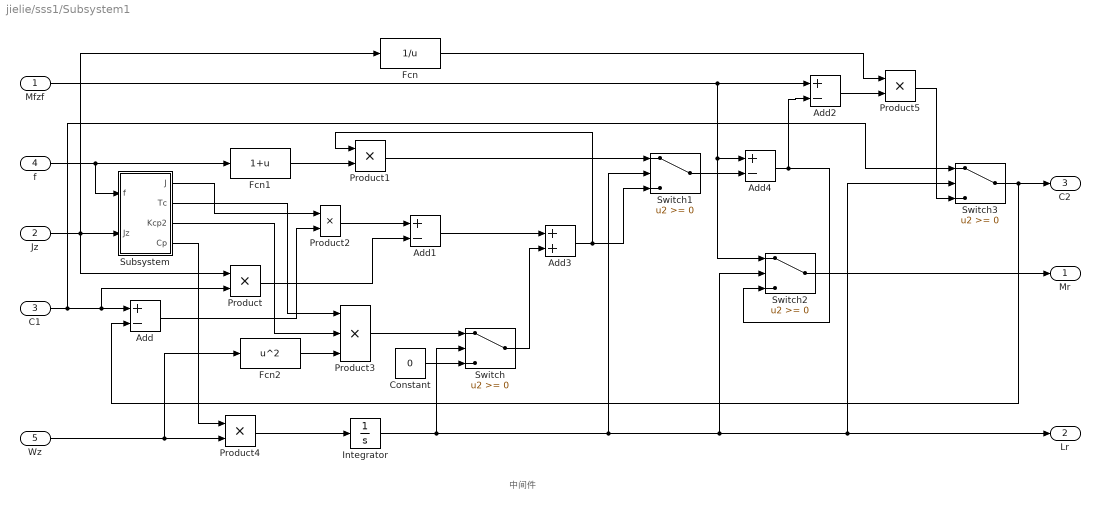
== system jielie/sss1/Subsystem1 ==
  note: 中间件
  Mfzf : Inport
  Jz : Inport  Port=2
  C1 : Inport  Port=3
  f : Inport  Port=4
  Wz : Inport  Port=5
  Add{,1..2,4} (4 alike) : Sum  Inputs=+-
  Add3 : Sum
  Constant : Constant  Value=0
  Fcn : Fcn  Expr=1/u
  Fcn1 : Fcn  Expr=1+u
  Fcn2 : Fcn  Expr=u^2
  Integrator : Integrator  LimitOutput=on  UpperSaturationLimit=15  LowerSaturationLimit=0
  Product{,1..2,4..5} (5 alike) : Product
  Product3 : Product  Inputs=3
  Subsystem : Subsystem
  Switch{,1..3} (4 alike) : Switch
  Mr : Outport
  Lr : Outport  Port=2
  C2 : Outport  Port=3
  wires:
  C1/1 -> Switch3/1, Product/2, Add/1
  f/1 -> Subsystem/1(f), Fcn1/1
  Fcn1/1 -> Product1/2
  Product1/1 -> Switch1/1
  Switch1/1 -> Add4/2
  Mfzf/1 -> Add2/1, Add4/1, Switch2/1
  Add2/1 -> Product5/2
  Fcn/1 -> Product5/1
  Switch2/1 -> Mr/1
  Add4/1 -> Add2/2, Switch2/3
  Jz/1 -> Product/1, Subsystem/2(Jz), Fcn/1
  Wz/1 -> Fcn2/1, Product4/2
  Fcn2/1 -> Product3/3
  Integrator/1 -> Lr/1, Switch3/2, Switch2/2, Switch1/2, Switch/2
  Product3/1 -> Switch/1
  Constant/1 -> Switch/3
  Add1/1 -> Add3/1
  Switch/1 -> Add3/2
  Add3/1 -> Product1/1, Switch1/3
  Product/1 -> Add1/2
  Product2/1 -> Add1/1
  Add/1 -> Product2/2
  Subsystem/4(Cp) -> Product4/1
  Subsystem/3(Kcp2) -> Product3/2
  Subsystem/1(J) -> Product2/1
  Subsystem/2(Tc) -> Product3/1
  Product4/1 -> Integrator/1
  Switch3/1 -> Add/2, C2/1
  Product5/1 -> Switch3/3

== system jielie/sss1/Subsystem2 ==
  note: 从动件
  Mr : Inport
  J2 : Inport  Port=2
  C2 : Inport  Port=3
  n2in : Inport  Port=4
  Add : Sum  Inputs=+-
  Add1 : Sum
  Fcn : Fcn  Expr=30*u/pi
  Integrator : Integrator
  Product : Product
  M2 : Outport
  n2 : Outport  Port=2
  wires:
  Mr/1 -> Add/1
  Add/1 -> M2/1
  J2/1 -> Product/1
  Integrator/1 -> Add1/1
  n2in/1 -> Add1/2
  Add1/1 -> n2/1
  Product/1 -> Add/2
  Fcn/1 -> Integrator/1
  C2/1 -> Fcn/1, Product/2

== system jielie/sss1/Subsystem3 ==
  note: 主动件
  M1 : Inport
  n1 : Inport  Port=2
  J1 : Inport  Port=3
  Derivative : Derivative
  Fcn2 : Fcn  Expr=u*pi/30
  Product : Product
  Sum : Sum  Inputs=|+-
  Mfzf : Outport
  wf : Outport  Port=2
  C1 : Outport  Port=3
  wires:
  n1/1 -> Fcn2/1
  Fcn2/1 -> wf/1, Derivative/1
  M1/1 -> Sum/1
  J1/1 -> Product/2
  Derivative/1 -> Product/1, C1/1
  Product/1 -> Sum/2
  Sum/1 -> Mfzf/1

== system jielie/sss2/Subsystem ==
  note: 阻尼系数模块
  J : Constant  Value=0.119507
  J2l : Constant  Value=0.092495
  Jk : Constant  Value=0.0694875
  f1 : Constant  Value=0.6
  J1 : Outport
  Jz : Outport  Port=2
  J2 : Outport  Port=3
  f : Outport  Port=4
  wires:
  J/1 -> J1/1
  Jk/1 -> Jz/1
  J2l/1 -> J2/1
  f1/1 -> f/1

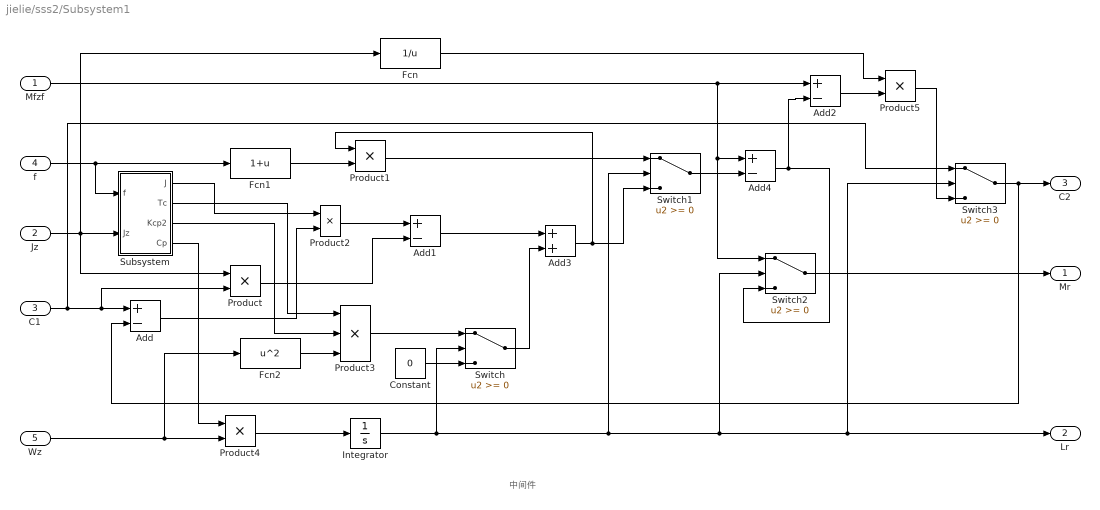
== system jielie/sss2/Subsystem1 ==
  note: 中间件
  Mfzf : Inport
  Jz : Inport  Port=2
  C1 : Inport  Port=3
  f : Inport  Port=4
  Wz : Inport  Port=5
  Add{,1..2,4} (4 alike) : Sum  Inputs=+-
  Add3 : Sum
  Constant : Constant  Value=0
  Fcn : Fcn  Expr=1/u
  Fcn1 : Fcn  Expr=1+u
  Fcn2 : Fcn  Expr=u^2
  Integrator : Integrator  LimitOutput=on  UpperSaturationLimit=15  LowerSaturationLimit=0
  Product{,1..2,4..5} (5 alike) : Product
  Product3 : Product  Inputs=3
  Subsystem : Subsystem
  Switch{,1..3} (4 alike) : Switch
  Mr : Outport
  Lr : Outport  Port=2
  C2 : Outport  Port=3
  wires:
  C1/1 -> Switch3/1, Product/2, Add/1
  f/1 -> Subsystem/1(f), Fcn1/1
  Fcn1/1 -> Product1/2
  Product1/1 -> Switch1/1
  Switch1/1 -> Add4/2
  Mfzf/1 -> Add2/1, Add4/1, Switch2/1
  Add2/1 -> Product5/2
  Fcn/1 -> Product5/1
  Switch2/1 -> Mr/1
  Add4/1 -> Add2/2, Switch2/3
  Jz/1 -> Product/1, Subsystem/2(Jz), Fcn/1
  Wz/1 -> Fcn2/1, Product4/2
  Fcn2/1 -> Product3/3
  Integrator/1 -> Lr/1, Switch3/2, Switch2/2, Switch1/2, Switch/2
  Product3/1 -> Switch/1
  Constant/1 -> Switch/3
  Add1/1 -> Add3/1
  Switch/1 -> Add3/2
  Add3/1 -> Product1/1, Switch1/3
  Product/1 -> Add1/2
  Product2/1 -> Add1/1
  Add/1 -> Product2/2
  Subsystem/4(Cp) -> Product4/1
  Subsystem/3(Kcp2) -> Product3/2
  Subsystem/1(J) -> Product2/1
  Subsystem/2(Tc) -> Product3/1
  Product4/1 -> Integrator/1
  Switch3/1 -> Add/2, C2/1
  Product5/1 -> Switch3/3

== system jielie/sss2/Subsystem2 ==
  note: 从动件
  Mr : Inport
  J2 : Inport  Port=2
  C2 : Inport  Port=3
  n2in : Inport  Port=4
  Add : Sum  Inputs=+-
  Add1 : Sum
  Fcn : Fcn  Expr=30*u/pi
  Integrator : Integrator
  Product : Product
  M2 : Outport
  n2 : Outport  Port=2
  wires:
  Mr/1 -> Add/1
  Add/1 -> M2/1
  J2/1 -> Product/1
  Integrator/1 -> Add1/1
  n2in/1 -> Add1/2
  Add1/1 -> n2/1
  Product/1 -> Add/2
  Fcn/1 -> Integrator/1
  C2/1 -> Fcn/1, Product/2

== system jielie/sss2/Subsystem3 ==
  note: 主动件
  M1 : Inport
  n1 : Inport  Port=2
  J1 : Inport  Port=3
  Derivative : Derivative
  Fcn2 : Fcn  Expr=u*pi/30
  Product : Product
  Sum : Sum  Inputs=|+-
  Mfzf : Outport
  wf : Outport  Port=2
  C1 : Outport  Port=3
  wires:
  n1/1 -> Fcn2/1
  Fcn2/1 -> wf/1, Derivative/1
  M1/1 -> Sum/1
  J1/1 -> Product/2
  Derivative/1 -> Product/1, C1/1
  Product/1 -> Sum/2
  Sum/1 -> Mfzf/1

== system jielie/ranqilunji1/diyawolun/turbine_TN ==
  Pi : Inport
  eta : Inport  Port=2
  Tin : Inport  Port=3
  Gin : Inport  Port=4
  Add : Sum  Inputs=-+
  Add1 : Sum  Inputs=-+
  Constant : Constant
  Fcn : Fcn  Expr=1/(u[1]^u[2])
  K2 : Subsystem
  Mux : Mux  Inputs=2
  Product : Product  Inputs=4  RndMeth=Zero
  Product1 : Product  RndMeth=Zero
  Product2 : Product  RndMeth=Zero
  m : Fcn  Expr=(u-1)/u
  Tout : Outport
  Nout : Outport  Port=2
  wires:
  Tin/1 -> K2/1(T1), Product1/2, Product/4
  Pi/1 -> Mux/1
  m/1 -> Mux/2
  Mux/1 -> Fcn/1
  Fcn/1 -> Add/1
  Add/1 -> Product2/2
  eta/1 -> Product2/1
  Product2/1 -> Add1/1, Product/1
  Constant/1 -> Add/2, Add1/2
  Product1/1 -> Tout/1
  Product/1 -> Nout/1
  Add1/1 -> Product1/1
  K2/2(Cp) -> Product/2
  Gin/1 -> Product/3
  K2/1(K) -> m/1

== system jielie/ranqilunji1/diyayaqiji/Subsystem1 ==
  Gin : Inport
  Pin : Inport  Port=2
  Tin : Inport  Port=3
  Divide : Product  Inputs=*/
  Divide1 : Product  Inputs=*/
  Divide2 : Product  Inputs=*/
  Fcn : Fcn  Expr=sqrt(u)
  P0 : Constant  Value=100000
  Product : Product  RndMeth=Zero
  T0 : Constant  Value=288
  Gz : Outport
  wires:
  Tin/1 -> Divide/1
  T0/1 -> Divide/2
  Divide/1 -> Fcn/1
  Pin/1 -> Divide1/1
  P0/1 -> Divide1/2
  Gin/1 -> Divide2/1
  Divide1/1 -> Divide2/2
  Fcn/1 -> Product/1
  Divide2/1 -> Product/2
  Product/1 -> Gz/1
